simulink model "doble_p"  (R2022b)
settings: Solver=VariableStepAuto  StartTime=0.0  StopTime=10  MaxStep=0.00001  RelTol=1e-3
values from neighbouring files (symbols this model uses):
  g = 9.81    [clase230123.m]
  l1 = 0.3    [clase230123.m]
  l2 = 0.25    [clase230123.m]
  m1 = 0.2    [clase230123.m]
  m2 = 0.1    [clase230123.m]
settings Model: Creator=mluser  LastModifiedBy=mluser

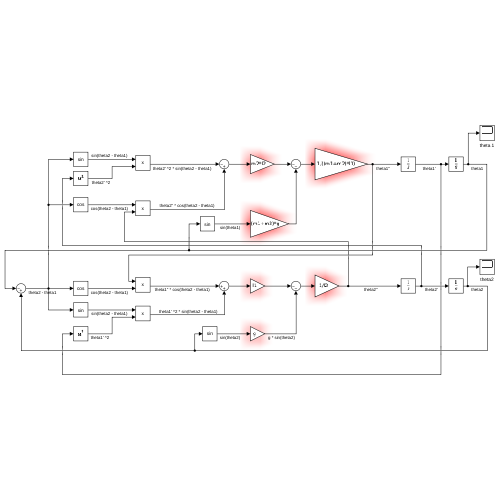
[thumbnail: Simulink's stored preview of the top-level diagram]
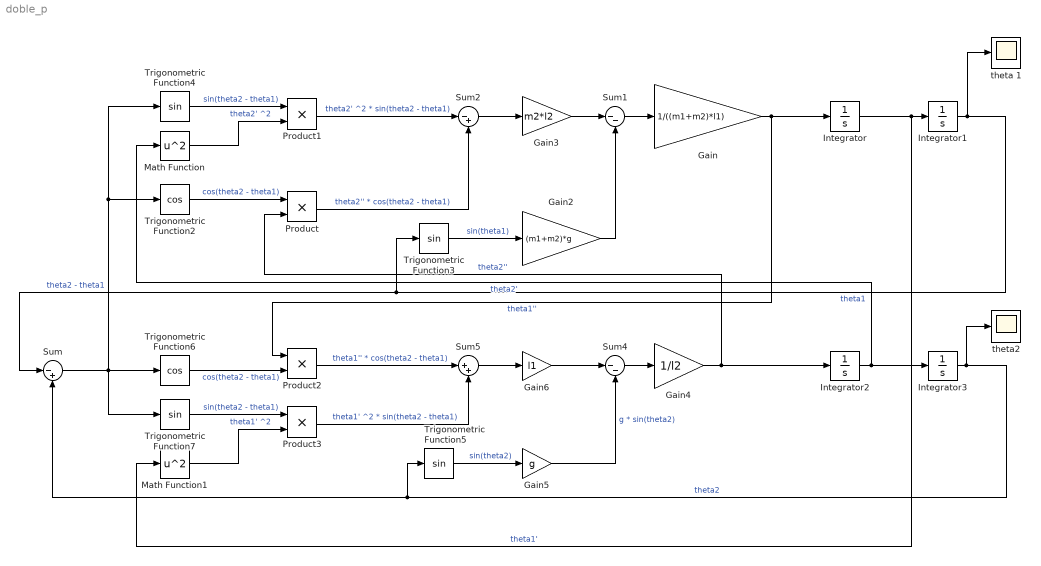
== system doble_p ==
  Gain : Gain  Gain=1/((m1+m2)*l1)
  Gain2 : Gain  Gain=(m1+m2)*g
  Gain3 : Gain  Gain=m2*l2
  Gain4 : Gain  Gain=1/l2
  Gain5 : Gain  Gain=g
  Gain6 : Gain  Gain=l1
  Integrator : Integrator
  Integrator1 : Integrator
  Integrator2 : Integrator
  Integrator3 : Integrator  InitialCondition=(35*pi)/180
  Math Function : Math  Operator=square
  Math Function1 : Math  Operator=square
  Product{,1..3} (4 alike) : Product
  Sum : Sum  Inputs=|-+
  Sum1 : Sum  Inputs=|--
  Sum2 : Sum  Inputs=|-+
  Sum4 : Sum  Inputs=|--
  Sum5 : Sum  Inputs=|++
  Trigonometric Function2 : Trigonometry  Operator=cos
  Trigonometric Function{3..5,7} (4 alike) : Trigonometry
  Trigonometric Function6 : Trigonometry  Operator=cos
  theta 1 : Scope
  theta2 : Scope
  wires:
  Sum1/1 -> Gain/1
  Gain3/1 -> Sum1/1
  Gain2/1 -> Sum1/2
  Trigonometric Function3/1 -> Gain2/1  "sin(theta1)"
  Sum2/1 -> Gain3/1
  Product/1 -> Sum2/2  "theta2'' * cos(theta2 - theta1)"
  Trigonometric Function2/1 -> Product/1  "cos(theta2 - theta1)"
  Product1/1 -> Sum2/1  "theta2' ^2 * sin(theta2 - theta1)"
  Math Function/1 -> Product1/2  "theta2' ^2"
  Trigonometric Function4/1 -> Product1/1  "sin(theta2 - theta1)"
  Gain/1 -> Product2/1, Integrator/1  "theta1''"
  Integrator/1 -> Math Function1/1, Integrator1/1  "theta1'"
  Integrator1/1 -> theta 1/1, Sum/1, Trigonometric Function3/1  "theta1"
  Sum4/1 -> Gain4/1
  Trigonometric Function5/1 -> Gain5/1  "sin(theta2)"
  Gain5/1 -> Sum4/2  "g * sin(theta2)"
  Gain6/1 -> Sum4/1
  Sum5/1 -> Gain6/1
  Product2/1 -> Sum5/1  "theta1'' * cos(theta2 - theta1)"
  Product3/1 -> Sum5/2  "theta1' ^2 * sin(theta2 - theta1)"
  Trigonometric Function6/1 -> Product2/2  "cos(theta2 - theta1)"
  Sum/1 -> Trigonometric Function4/1, Trigonometric Function2/1, Trigonometric Function7/1, Trigonometric Function6/1  "theta2 - theta1"
  Trigonometric Function7/1 -> Product3/1  "sin(theta2 - theta1)"
  Math Function1/1 -> Product3/2  "theta1' ^2"
  Gain4/1 -> Product/2, Integrator2/1  "theta2''"
  Integrator2/1 -> Math Function/1, Integrator3/1  "theta2'"
  Integrator3/1 -> theta2/1, Sum/2, Trigonometric Function5/1  "theta2"
